simulink model "ctrl_custom_2016"  (R2019b)
settings: Solver=ode4  StartTime=0.0  StopTime=inf  FixedStep=0.01  RelTol=1e-3  EnableMultiTasking=on
values from neighbouring files (symbols this model uses):
  B = [zeros(3); inv(M); zeros(3)]    [ctrl_custom_init.m]
  D = reshape([abs(u).*(-3.545e-1)+u.^2.*3.787+6.555e-1,0.0,0.0,0.0,t2.*(1.61e2./2.0e2)+t3.*(3.47e2./1.25e2)+v.^2.*6.491e1+1.33e2./1.0e2,t2.*(-1.3e1./1.0e2)+t3.*2.088e-1,0.0,t2.*(6.9e1./2.0e1)+t3.*(1.69e2./2.0e2)+2.9e1./4.0,t2.*(3.0./4.0)-t3.*(2.0./2.5e1)+1.9e1./1.0e1],[3,3])    [D.m]    (also in ctrl_custom_init.m = [)
  L1 = diag([1 1 1])    [ctrl_custom_init.m]
  L2 = diag([0.1 0.1 0.1])    [ctrl_custom_init.m]
  L3 = diag([0.025 0.01 0.0001])    [ctrl_custom_init.m]
  M = [ ... (first row only)    [ctrl_custom_init.m]
  x_init = zeros(1,9)    [ctrl_custom_init.m]
libraries: simulink x1
(part 2 of 2)

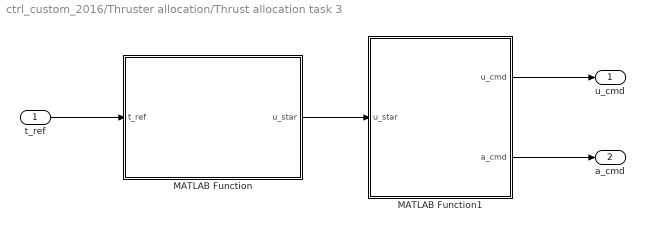
== system ctrl_custom_2016/Thruster allocation/Thrust allocation task 3 ==
  t_ref : Inport
  MATLAB Function : MATLAB Function  TreatAsAtomicUnit=on
  MATLAB Function1 : MATLAB Function  TreatAsAtomicUnit=on
  u_cmd : Outport
  a_cmd : Outport  Port=2
  wires:
  MATLAB Function1/2(a_cmd) -> a_cmd/1
  MATLAB Function1/1(u_cmd) -> u_cmd/1
  MATLAB Function/1(u_star) -> MATLAB Function1/1(u_star)
  t_ref/1 -> MATLAB Function/1(t_ref)

== matlab function ctrl_custom_2016/Thruster allocation/Thrust allocation task 2/MATLAB Function ==
  data: t_ref input; u_star output; angles input
function u_star = thrust_allocation_2(t_ref, angles)
% Calculates thrust and vsp angles for set angles

% Parameters
lx_1 = 0.3875;
lx_2 = -0.4574;
ly_1 = 0.055;
ly_2 = -0.055;

K1 = 1.03;
K2 = K1;
K3 = 2.629;

a1 = angles(1);
a2 = angles(2);

B = [cos(a1) cos(a2) 0; 
    sin(a1) sin(a2) 1; 
    lx_2*sin(a1)-ly_1*cos(a2) lx_2*sin(a2)-ly_2*cos(a2) lx_1];
K = diag([K1, K2, K3]);

% Calculate u with pseudo inverse method
u_star = pinv(B*K) * t_ref;

end

== matlab function ctrl_custom_2016/Thruster allocation/Thrust allocation task 2/MATLAB Function1 ==
  data: u_star input; u_cmd output; a input; a_cmd output
function [u_cmd, a_cmd] = beta_procedure(u_star, a)
% Flips angle and thrust if thrust is negative

% initialize outputs
u_cmd = [0 0 0]';
a_cmd = [0 0]';

if u_star(1) < 0
    % flip thrust
    u_cmd(1) = - u_star(1);
    
    % flip angle
    if a(1) < 0
        a_cmd(1) = a(1) + pi;
    else
        a_cmd(1) = a(1) - pi;
    end
else
    a_cmd(1) = a(1);
    u_cmd(1) = u_star(1);
end
    
if u_star(2) < 0
    % flip thrust
    u_cmd(2) = - u_star(2);
    
    % flip angle
    if a(2) < 0
        a_cmd(2) = a(2) + pi;
    else
        a_cmd(2) = a(2) - pi;
    end
else
    a_cmd(2) = a(2);
    u_cmd(2) = u_star(2);
end

u_cmd(3) = u_star(3);
    
end

== matlab function ctrl_custom_2016/Thruster allocation/Thrust allocation task 3/MATLAB Function ==
  data: t_ref input; u_star output
function u_star = thrust_allocation_3(t_ref)

% parameters
lx_1 = 0.3875;
lx_2 = -0.4574;
ly_1 = 0.055;
ly_2 = -0.055;

K1 = 1.03;
K2 = K1;
K3 = 2.629;

K = diag([K1, K1, K2, K2, K3]);
B = [
    1 0 1 0 0;
    0 1 0 1 1;
    ly_1 lx_2 ly_2 lx_2 lx_1;
];

% Calculate thrust cmd using pseude inverse method
u_star = pinv(B*K)*t_ref;

end

== matlab function ctrl_custom_2016/Thruster allocation/Thrust allocation task 3/MATLAB Function1 ==
  data: u_star input; u_cmd output; a_cmd output
function [u_cmd, a_cmd] = gamma_procedure(u_star)
% param u_decomposed = [u1_x, u1_y, u2_x, u2_y, u3]
% this function maps u_decomposed to its thruster input and angles

% TODO: limit output u to [0,1]?

% initialize output values
u_cmd = [0 0 0]';
a_cmd = [0 0]';

u1_x = u_star(1);
u1_y = u_star(2);
u2_x = u_star(3);
u2_y = u_star(4);
u_cmd(3) = u_star(5);

a_cmd(1) = atan2(u1_y, u1_x);
a_cmd(2) = atan2(u2_y, u2_x);

u_cmd(1) = norm([u1_x, u1_y]);
u_cmd(2) = norm([u2_x, u2_y]);

end

== matlab function ctrl_custom_2016/Oberserver/MATLAB Function ==
  data: x_hat input; result output; D input; M input
function result = f_A(x_hat, D, M)

% Define the rotation matrix R
psi = x_hat(3);
R = [
    [cos(psi) -sin(psi) 0];
    [sin(psi) cos(psi) 0];
    [0 0 1]
];

% define system matrix A
A = [
    [zeros(3) R zeros(3)];
    [zeros(3) -M\D M\R'];
    [zeros(3,9)];
];

result = A*x_hat;

== matlab function ctrl_custom_2016/Pose1/MATLAB Function ==
  data: deg input; rad output
function rad = map_deg2rad(deg)
% maps deg in [-180,180] to rad in (-pi, pi]

rad = deg2rad(deg);

if rad <= -pi
    rad = 2*pi - rad;
elseif rad > pi
    rad = rad - 2*pi;
end

end

== matlab function ctrl_custom_2016/MATLAB Function ==
  data: btn input; signal output; signal input
function signal = switch_signal(btn, signal)

 if btn
     if signal
         signal = 0;
     else
         signal = 1;
     end
 end
 
 
end

== matlab function ctrl_custom_2016/MATLAB Function1 ==
  data: x_ned input; x_body output; psi input
function x_body = R_NED_BODY(x_ned, psi)

R = [
    [cos(psi) -sin(psi) 0];
    [sin(psi) cos(psi) 0];
    [0 0 1]
];

x_body = R'*x_ned;

== matlab function ctrl_custom_2016/Oberserver/MATLAB Function1 ==
  data: L1 input; L2 input; L3 input; M input; psi input; eta_diff input; result output
function result = f_L(L1, L2, L3, M, psi, eta_diff)

% Define the rotation matrix R
R = [
    [cos(psi) -sin(psi) 0];
    [sin(psi) cos(psi) 0];
    [0 0 1]
];

L = [L1; M\R'*L2; L3];

result = L*eta_diff;

== matlab function ctrl_custom_2016/Oberserver/MATLAB Function2 ==
  data: previous_measurements input; previous_measurements_new output; eta_measured input; signal_available input; eta_output output; eta_estimated input
function [previous_measurements_new, eta_output] = signal_check(previous_measurements, eta_measured, signal_available, eta_estimated)

if signal_available
    
    % check if signal has stalled
    has_stalled = true;
    for i=1:3
       if eta_measured ~= previous_measurements(i)
           has_stalled = false;
           break
       end
    end
    
    % determine output
    if has_stalled
        eta_output = eta_estimated;
    else
        eta_output = eta_measured;
    end
   
else
   eta_output = eta_estimated; 
end

% update previous measurements
previous_measurements_new = circshift(previous_measurements, 1, 2);
previous_measurements_new(:,1) = eta_measured;
   
end
